simulink model "playback_data"  (R2015a)
settings: Solver=FixedStepDiscrete  SolverMode=SingleTasking  StartTime=76  StopTime=110  FixedStep=sample_time  RelTol=1e-3
undefined symbols (not defined in the file): A1_notch_f1, A2_notch_f1, A_kalman_swing_load, A_kalman_transverse, A_kalman_vertical, A_lpf_accelerometer, A_lpf_dtau, A_lpf_fourbar_angles, A_lpf_imu, A_lpf_lateral_angle, B1_lpf_accelerometer, B1_lpf_dtau, B1_lpf_fourbar_angles, B1_lpf_imu, B1_lpf_lateral_angle, B1_notch_f1, B2_lpf_accelerometer, B2_lpf_dtau, B2_lpf_fourbar_angles, B2_lpf_imu, B2_lpf_lateral_angle, B2_notch_f1, B_dx_versus_x0, B_kalman_swing_load, B_kalman_transverse, B_kalman_vertical, backwards_K_sag_of_t, backwards_P_sag_of_t, C_kalman_swing_load, C_kalman_transverse, C_kalman_vertical, com_leg_motor, com_torso, contact_threshold, control_start_time, d_ankle_to_foot, d_vertical_com, desired_com_forward_velocity, desired_com_lateral_velocity, desired_initial_leg_roll_left, desired_initial_leg_roll_right, desired_stance_beta2, desired_standing_torso_pitch, desired_standing_torso_roll, desired_standing_z, desired_torso_pitch, desired_torso_roll, Discrete, enable_bouncing, fcut_contact, fdesignblkfcn, forward_dx_of_dxstar, forward_x_of_dxstar, g, gcbh, HIP_MTR_MAX_CONT_TORQUE, HIP_MTR_MAX_TORQUE, i_leg_motor, i_robot, i_torso ... (+78)
libraries: simulink x65, dsparch4 x18, ctrlSharedLib x14, dspfdesign x4
(part 5 of 13)

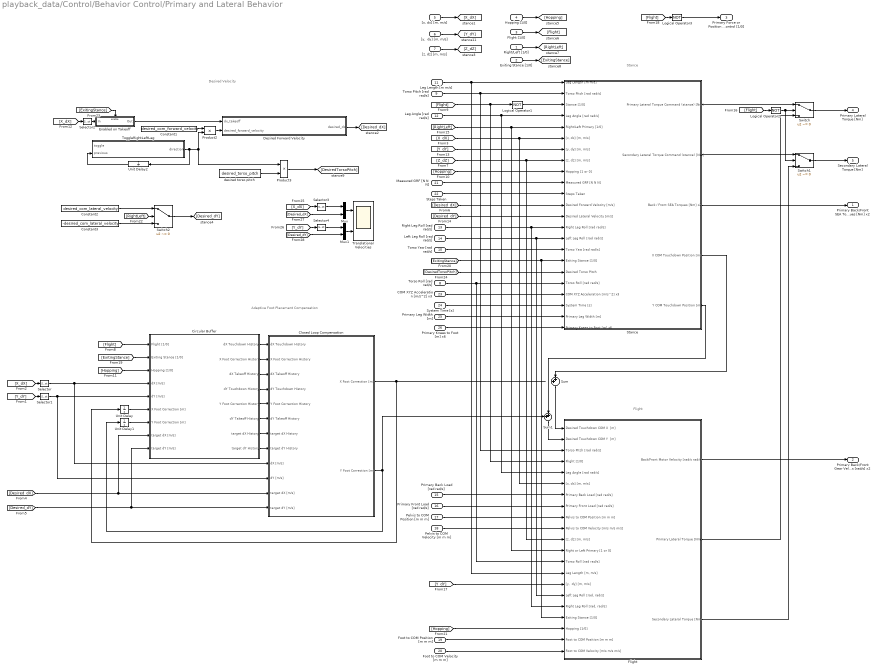
== system playback_data/Control/Behavior Control/Primary and Lateral Behavior ==
  note: Stance
  note: Flight
  note: Adaptive Foot Placement Compensation
  note: Desired Velocity
  Right/Left [1/0] : Inport
  Exiting Stance [1/0] : Inport  Port=2
  Flight [1/0] : Inport  Port=3
  Hopping [1/0] : Inport  Port=4
  "[x, dx] [m, m/s]" : Inport  Port=5
  "[y,  dy] [m, m/s]" : Inport  Port=6
  "[z, dz] [m, m/s]" : Inport  Port=7
  Torso Roll [rad rad/s] : Inport  Port=8
  Torso Pitch [rad rad/s] : Inport  Port=9
  Torso Yaw [rad rad/s] : Inport  Port=10
  Leg Length [m m/s] : Inport  Port=11
  Leg Angle [rad rad/s] : Inport  Port=12
  Right Leg Roll [rad rad/s] : Inport  Port=13
  Left Leg Roll [rad rad/s] : Inport  Port=14
  Primary Back Load [rad rad/s] : Inport  Port=15
  Primary Front Load [rad rad/s] : Inport  Port=16
  Pelvis to COM Position [m m m] : Inport  Port=17
  Pelvis to COM Velocity [m m m] : Inport  Port=18
  Foot to COM Position [m m m] : Inport  Port=19
  Foot to COM Velocity [m m m] : Inport  Port=20
  Measured GRF [N N N] : Inport  Port=21
  Steps Taken : Inport  Port=22
  COM XYZ Acceleration [m/s^2] x3 : Inport  Port=23
  System Time [s] : Inport  Port=24
  Primary Leg Width [m] : Inport  Port=25
  Primary Knees to Foot [m] x6 : Inport  Port=26
  Circular Buffer : Subsystem
  Closed Loop Compensation : Subsystem
  Constant1 : Constant  Value=desired_com_forward_velocity
  Constant2 : Constant  Value=desired_com_lateral_velocity
  Constant3 : Constant  Value=-desired_com_lateral_velocity
  Desired Forward Velocity : MATLAB Function  TreatAsAtomicUnit=on
  Enabled on Takeoff : Subsystem  TreatAsAtomicUnit=on
  Flight : Subsystem
  Logical Operator1 : Logic  Operator=NOT  AllPortsSameDT=off  OutDataTypeStr=boolean
  Logical Operator2 : Logic  Operator=NOT  AllPortsSameDT=off  OutDataTypeStr=boolean
  Logical Operator3 : Logic  Operator=NOT  AllPortsSameDT=off  OutDataTypeStr=boolean
  Mux : Mux  Inputs=2
  Mux1 : Mux  Inputs=2
  Product2 : Product
  Product3 : Product
  Selector{,1..4} (5 alike) : Selector  InputPortWidth=2  Indices=[2]
  Stance : Subsystem
  Sum : Sum  Inputs=++|
  Sum1 : Sum  Inputs=++|
  Switch : Switch  Criteria=u2 ~= 0
  Switch1 : Switch  Criteria=u2 ~= 0
  Switch2 : Switch  Criteria=u2 ~= 0
  ToggleRightLeftLeg : MATLAB Function  TreatAsAtomicUnit=on
      settings: MinAlgLoopOccurrences=on
  Translational Velocities : Scope  NumInputPorts=2
      settings: YMin=-1000~-5  YMax=1000~5  SaveName=ScopeData2  SampleInput=on
  Unit Delay : UnitDelay  SampleTime=-1
  Unit Delay1 : UnitDelay  SampleTime=-1
  Unit Delay2 : UnitDelay  InitialCondition=1  SampleTime=sample_time
  desired torso pitch : Constant  Value=desired_torso_pitch
  Primary Back/Front SEA Torques [Nm] x2 : Outport
  Primary Back/Front Gear Velocities [rad/s] x2 : Outport  Port=2
  Primary Force or Position Control [1/0] : Outport  Port=3  OutDataTypeStr=boolean
  Primary Lateral Torque [Nm] : Outport  Port=4
  Secondary Lateral Torque [Nm] : Outport  Port=5
  wires:
  Leg Length [m m/s]/1 -> Stance/1(Leg Length [m m/s]), Flight/14("Leg Length [m, m/s]")
  Torso Pitch [rad rad/s]/1 -> Stance/2(Torso Pitch [rad rad/s]), Flight/3(Torso Pitch [rad rad/s])
  [Hopping] -> Stance/9(Hopping [1 or 0])
  [X_dX] -> Flight/6("[x, dx] [m, m/s]"), Stance/6("[x, dx] [m, m/s]")
  [RightLeft] -> Flight/12(Right or Left Primary [1 or 0]), Stance/5(Right/Left Primary [1/0])
  Primary Back Load [rad rad/s]/1 -> Flight/7(Primary Back Load [rad rad/s])
  Primary Front Load [rad rad/s]/1 -> Flight/8(Primary Front Load [rad rad/s])
  Leg Angle [rad rad/s]/1 -> Flight/5(Leg Angle [rad rad/s]), Stance/4(Leg Angle [rad rad/s])
  Flight/1(Back/Front Motor Velocity [rad/s rad/s]) -> Primary Back/Front Gear Velocities [rad/s] x2/1
  Logical Operator1/1 -> Stance/3(Stance [1/0])
  [Flight] -> Circular Buffer/1(Flight [1/0])
  Pelvis to COM Position [m m m]/1 -> Flight/9(Pelvis to COM Position [m m m])
  [Z_dZ] -> Stance/8("[z, dz] [m, m/s]"), Flight/11("[z, dz] [m, m/s]")
  Pelvis to COM Velocity [m m m]/1 -> Flight/10(Pelvis to COM Velocity [m/s m/s m/s])
  Torso Roll [rad rad/s]/1 -> Flight/13(Torso Roll [rad rad/s]), Stance/19(Torso Roll [rad rad/s])
  Measured GRF [N N N]/1 -> Stance/10(Measured GRF [N N N])
  Steps Taken/1 -> Stance/11(Steps Taken)
  [Y_dY] -> Flight/15("[y,  dy] [m, m/s]")
  Circular Buffer/1("dX Touchdown History ") -> Closed Loop Compensation/1(dX Touchdown History)
  Circular Buffer/2(X Foot Correction History) -> Closed Loop Compensation/2(X Foot Correction History)
  Circular Buffer/3(dX Takeoff History) -> Closed Loop Compensation/3(dX Takeoff History)
  Circular Buffer/4("dY Touchdown History ") -> Closed Loop Compensation/4(dY Touchdown History)
  Circular Buffer/5(Y Foot Correction History) -> Closed Loop Compensation/5(Y Foot Correction History)
  Circular Buffer/6(dY Takeoff History) -> Closed Loop Compensation/6(dY Takeoff History)
  Circular Buffer/8(target dY History) -> Closed Loop Compensation/8(target dY History)
  Circular Buffer/7(target dX History) -> Closed Loop Compensation/7(target dX History)
  [Desired_dX] -> Circular Buffer/8(target dX [m/s]), Closed Loop Compensation/11(target dX [m/s])
  [Desired_dY] -> Circular Buffer/9(target dY [m/s]), Closed Loop Compensation/12("target dY [m/s] ")
  Stance/4(X COM Touchdown Position [m]) -> Sum/2
  Sum/1 -> Flight/1(Desired Touchdown COM X  [m])
  Closed Loop Compensation/1(X Foot Correction [m]) -> Unit Delay/1
  Selector1/1 -> Circular Buffer/5(dY [m/s]), Closed Loop Compensation/10(dY [m/s])
  Selector/1 -> Circular Buffer/4(dX [m/s]), Closed Loop Compensation/9(dX [m/s])
  Unit Delay1/1 -> Circular Buffer/7(Y Foot Correction [m])
  Unit Delay/1 -> Circular Buffer/6(X Foot Correction [m])
  Closed Loop Compensation/2(Y Foot Correction [m]) -> Unit Delay1/1, Sum1/1
  "[x, dx] [m, m/s]"/1 -> [X_dX]
  "[z, dz] [m, m/s]"/1 -> [Z_dZ]
  "[y,  dy] [m, m/s]"/1 -> [Y_dY]
  [X_dX] -> Selector/1
  [Y_dY] -> Selector1/1
  [Desired_dX] -> Stance/12(Desired Forward Velocity [m/s])
  Flight [1/0]/1 -> [Flight]
  [Flight] -> Flight/4(Flight [1/0]), Logical Operator1/1
  Hopping [1/0]/1 -> [Hopping]
  Stance/5(Y COM Touchdown Position [m]) -> Sum1/2
  Sum1/1 -> Flight/2(Desired Touchdown COM Y  [m])
  Right Leg Roll [rad rad/s]/1 -> Flight/17("Right Leg Roll [rad, rad/s]"), Stance/14(Right Leg Roll [rad rad/s])
  Left Leg Roll [rad rad/s]/1 -> Flight/16("Left Leg Roll [rad, rad/s]"), Stance/15(Left Leg Roll [rad rad/s])
  [Y_dY] -> Stance/7("[y, dy] [m, m/s]")
  [Desired_dY] -> Stance/13(Desired Lateral Velocity [m/s])
  Right/Left [1/0]/1 -> [RightLeft]
  Logical Operator2/1 -> Switch1/2, Switch/2
  Flight/2(Primary Lateral Torque [Nm]) -> Switch/3
  Flight/3(Secondary Lateral Torque [Nm]) -> Switch1/3
  [Flight] -> Logical Operator2/1
  Switch/1 -> Primary Lateral Torque [Nm]/1
  Switch1/1 -> Secondary Lateral Torque [Nm]/1
  [Flight] -> Logical Operator3/1
  Logical Operator3/1 -> Primary Force or Position Control [1/0]/1
  Torso Yaw [rad rad/s]/1 -> Stance/16(Torso Yaw [rad rad/s])
  [Hopping] -> Circular Buffer/3(Hopping [1/0])
  [ExitingStance] -> Circular Buffer/2(Exiting Stance [1/0])
  Exiting Stance [1/0]/1 -> [ExitingStance]
  [ExitingStance] -> Flight/18(Exiting Stance [1/0]), Stance/17(Exiting Stance [1/0])
  [Hopping] -> Flight/19(Hopping [1/0])
  [X_dX] -> Selector2/1
  Switch2/1 -> [Desired_dY]
  Enabled on Takeoff/1(Out) -> Desired Forward Velocity/1(dx_takeoff)
  [RightLeft] -> Switch2/2
  Constant2/1 -> Switch2/1
  Constant3/1 -> Switch2/3
  [ExitingStance] -> Enabled on Takeoff/Enable
  Selector2/1 -> Enabled on Takeoff/1(In)
  Desired Forward Velocity/1(desired_dx) -> [Desired_dX]
  Product2/1 -> Desired Forward Velocity/2(desired_forward_velocity)
  ToggleRightLeftLeg/1(direction) -> Product2/2, Product3/1, Unit Delay2/1
  Unit Delay2/1 -> ToggleRightLeftLeg/2(previous)
  Constant1/1 -> Product2/1
  desired torso pitch/1 -> Product3/2
  Product3/1 -> [DesiredTorsoPitch]
  [DesiredTorsoPitch] -> Stance/18(Desired Torso Pitch)
  Foot to COM Position [m m m]/1 -> Flight/20(Foot to COM Position [m m m])
  Foot to COM Velocity [m m m]/1 -> Flight/21(Foot to COM Velocity [m/s m/s m/s])
  [X_dX] -> Selector3/1
  Selector3/1 -> Mux/1
  [Y_dY] -> Selector4/1
  Selector4/1 -> Mux1/1
  Mux/1 -> Translational Velocities/1
  Mux1/1 -> Translational Velocities/2
  [Desired_dY] -> Mux1/2
  [Desired_dX] -> Mux/2
  COM XYZ Acceleration [m/s^2] x3/1 -> Stance/20(COM XYZ Acceleration [m/s^2] x3)
  System Time [s]/1 -> Stance/21(System Time [s])
  Primary Leg Width [m]/1 -> Stance/22(Primary Leg Width [m])
  Stance/2(Secondary Lateral Torque Command (stance) [Nm]) -> Switch1/1
  Stance/3(Back / Front SEA Torques [Nm] x2) -> Primary Back/Front SEA Torques [Nm] x2/1
  Stance/1(Primary Lateral Torque Command (stance) [Nm]) -> Switch/1
  Primary Knees to Foot [m] x6/1 -> Stance/23(Primary Knees to Foot [m] x6)

== system playback_data/Control/Behavior Control/R Leg Calculator ==
  Front [rad rad/s] : Inport
  Back [rad rad/s] : Inport  Port=2
  Constant : Constant  Value=d_ankle_to_foot-0.01
  Demux1 : Demux  Outputs=2
  Gain1 : Gain  Gain=2*l_seg
  Gain2 : Gain  Gain=l_seg
  Gain3 : Gain  Gain=-1
  Gain4 : Gain  Gain=0.5
  Gain5 : Gain  Gain=0.5
  Gain6 : Gain  Gain=2
  Mux1 : Mux  Inputs=2
  Product : Product  RndMeth=Zero
  Sum : Sum  Inputs=++|
  Sum4 : Sum  Inputs=+|+
  Sum5 : Sum  Inputs=+|-
  Trigonometric Function : Trigonometry  Operator=cos
  Trigonometric Function1 : Trigonometry
  "Leg Length [m m/s] " : Outport
  Leg Angle [rad rad/s] : Outport  Port=2
  Leg Splay [rad rad/s] : Outport  Port=3
  w [m] : Outport  Port=4
  wires:
  Constant/1 -> Sum/1
  Sum/1 -> Mux1/1
  Gain6/1 -> w [m]/1
  Gain4/1 -> Trigonometric Function1/1, Trigonometric Function/1
  Trigonometric Function/1 -> Gain1/1
  Gain1/1 -> Sum/2
  Trigonometric Function1/1 -> Gain2/1
  Product/1 -> Mux1/2
  Front [rad rad/s]/1 -> Sum5/2, Sum4/2
  Back [rad rad/s]/1 -> Sum4/1, Sum5/1
  Demux1/2 -> Gain3/1
  Gain3/1 -> Product/2
  Demux1/1 -> Gain4/1
  Gain2/1 -> Product/1, Gain6/1
  Sum5/1 -> Leg Splay [rad rad/s]/1, Demux1/1
  Mux1/1 -> "Leg Length [m m/s] "/1
  Sum4/1 -> Gain5/1
  Gain5/1 -> Leg Angle [rad rad/s]/1

== system playback_data/Control/Behavior Control/Secondary Leg Behavior ==
  note: Mirror the primary
      | leg motion
  note: Position control the
      | individual four bar segments
  note: Convert to
      | four-bar angles
  Secondary Back Load [rad rad/s] : Inport
  Secondary Front Load [rad rad/s] : Inport  Port=2
  Torso Pitch [rad rad/s] : Inport  Port=3
  Primary Leg Angle [rad rad/s] : Inport  Port=4
  Primary Leg Length [m m/s] : Inport  Port=5
  Avoid Hitting Mechanical Limits : MATLAB Function  TreatAsAtomicUnit=on
  Back/Front PD : Subsystem
  Constant4 : Constant  Value=0
  Demux{1..3,5} (4 alike) : Demux  Outputs=2
  Demux6 : Demux  Outputs=6
  Fcn2 : Fcn  Expr=2*pi-u(1)
  Lowpass Filter (Swing) : Subsystem  DialogController=fdesignblkfcn  InitFcn=fdesignblkfcn(gcbh, {'InitFcn'});  mask(Lowpass Filter){}
      mask help: Design a lowpass filter
      settings: CopyFcn=fdesignblkfcn(gcbh, {'CopyFcn'});
      mask Help: helpview(mapfilelocation('dsp'), 'dsplowpassfilter');
      mask Display: disp('Lowpass')
  Mirrored Leg Length Target : MATLAB Function  TreatAsAtomicUnit=on
  Mux{1..4,7,11} (6 alike) : Mux  Inputs=2
  Mux5 : Mux  Inputs=3
  Mux6 : Mux  Inputs=3
  Sum : Sum  Inputs=++|
  Terminator : Terminator
  Virtual Leg to Four Bar : MATLAB Function  TreatAsAtomicUnit=on
  k_virtual1 : Gain  Gain=2
  k_virtual6 : Gain  Gain=-1
  Secondary Back/Front Motor Torque [Nm Nm] : Outport
  wires:
  Demux5/1 -> Fcn2/1
  Mirrored Leg Length Target/2(dl_leg) -> Mux5/2
  Mirrored Leg Length Target/3(ddl_leg) -> Mux5/3
  Mirrored Leg Length Target/1(l_leg) -> Mux5/1
  Constant4/1 -> Mux6/3
  k_virtual6/1 -> Mux6/2
  Fcn2/1 -> Mux6/1
  Mux7/1 -> Demux6/1
  Virtual Leg to Four Bar/1(back) -> Avoid Hitting Mechanical Limits/1(back_desired)
  Virtual Leg to Four Bar/2(dback) -> Avoid Hitting Mechanical Limits/2(dback_desired)
  Virtual Leg to Four Bar/3(ddback) -> Avoid Hitting Mechanical Limits/3(ddback_desired)
  Virtual Leg to Four Bar/4(front) -> Avoid Hitting Mechanical Limits/4(front_desired)
  Virtual Leg to Four Bar/5(dfront) -> Avoid Hitting Mechanical Limits/5(dfront_desired)
  Virtual Leg to Four Bar/6(ddfront) -> Avoid Hitting Mechanical Limits/6(ddfront_desired)
  Demux6/1 -> Virtual Leg to Four Bar/1(l_leg)
  Demux6/2 -> Virtual Leg to Four Bar/2(dl_leg)
  Demux6/3 -> Virtual Leg to Four Bar/3(ddl_leg)
  Demux6/4 -> Virtual Leg to Four Bar/4(phi)
  Demux6/5 -> Virtual Leg to Four Bar/5(dphi)
  Demux6/6 -> Virtual Leg to Four Bar/6(ddphi)
  Mux11/1 -> Back/Front PD/4(Measured Velocity [rad/s] [back front])
  Demux2/2 -> Mux11/2
  Mux4/1 -> Back/Front PD/3(Measured Position [rad] [back front])
  Mux1/1 -> Back/Front PD/1(Desired Position [rad] [back front])
  Demux3/2 -> Mux11/1
  Demux3/1 -> Mux4/1
  Avoid Hitting Mechanical Limits/2(front_cmd) -> Mux1/2
  Avoid Hitting Mechanical Limits/1(back_cmd) -> Mux1/1
  Demux2/1 -> Mux4/2
  Secondary Front Load [rad rad/s]/1 -> Demux2/1
  Secondary Back Load [rad rad/s]/1 -> Demux3/1
  Avoid Hitting Mechanical Limits/3(dback_cmd) -> Mux2/1
  Avoid Hitting Mechanical Limits/4(dfront_cmd) -> Mux2/2
  Avoid Hitting Mechanical Limits/5(ddback_cmd) -> Mux3/1
  Avoid Hitting Mechanical Limits/6(ddfront_cmd) -> Mux3/2
  Mux2/1 -> Back/Front PD/2(Desired Velocity [rad/s] [back front])
  Primary Leg Angle [rad rad/s]/1 -> Sum/2
  Demux1/1 -> Mirrored Leg Length Target/1(primary_l_leg)
  Demux1/2 -> Mirrored Leg Length Target/2(primary_dl_leg)
  Primary Leg Length [m m/s]/1 -> Demux1/1
  Sum/1 -> Demux5/1
  Torso Pitch [rad rad/s]/1 -> k_virtual1/1
  k_virtual1/1 -> Sum/1
  Mux5/1 -> Mux7/1
  Mux3/1 -> Terminator/1
  Demux5/2 -> k_virtual6/1
  Mux6/1 -> Mux7/2
  Back/Front PD/1(Commanded Velocity [rad/s] [back front]) -> Lowpass Filter (Swing)/1(In)
  Lowpass Filter (Swing)/1(Out) -> Secondary Back/Front Motor Torque [Nm Nm]/1

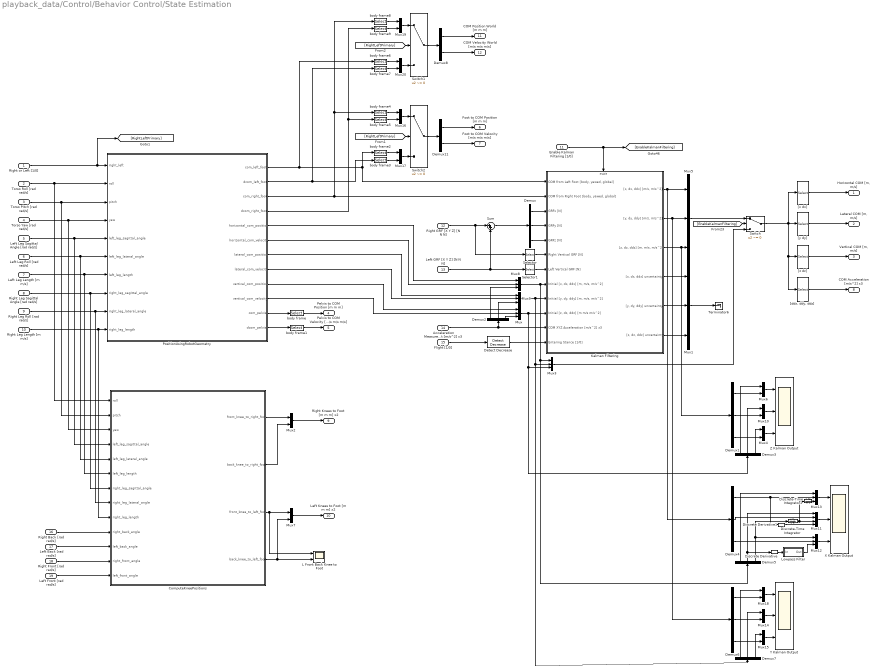
== system playback_data/Control/Behavior Control/State Estimation ==
  Right or Left [1/0] : Inport
  Torso Roll [rad rad/s] : Inport  Port=2
  Torso Pitch [rad rad/s] : Inport  Port=3
  Torso Yaw [rad rad/s] : Inport  Port=4
  Left Leg Sagittal Angle [rad rad/s] : Inport  Port=5
  Left Leg Roll [rad rad/s] : Inport  Port=6
  Left Leg Length [m m/s] : Inport  Port=7
  Right Leg Sagittal Angle [rad rad/s] : Inport  Port=8
  Right Leg Roll [rad rad/s] : Inport  Port=9
  Right Leg Length [m m/s] : Inport  Port=10
  Enable Kalman Filtering [1/0] : Inport  Port=11
  Right GRF [X Y Z] [N N N] : Inport  Port=12
  Left GRF [X Y Z] [N N N] : Inport  Port=13
  " Acceleration Measurement [m/s^2] x3" : Inport  Port=14
  Flight [1/0] : Inport  Port=15
  Right Back [rad rad/s] : Inport  Port=16
  Left Back [rad rad/s] : Inport  Port=17
  Right Front [rad rad/s] : Inport  Port=18
  Left Front [rad rad/s] : Inport  Port=19
  ComputeKneePositions : MATLAB Function  TreatAsAtomicUnit=on
  Demux{,1..7} (8 alike) : Demux  Outputs=3
  Demux11 : Demux  Outputs=2
  Demux8 : Demux  Outputs=2
  Detect Decrease : simulink/Logic and Bit Operations/Detect Decrease  vinit=0.0  InputProcessing=Inherited  OutDataTypeStr=boolean
  Discrete Derivative : simulink/Discrete/Discrete Derivative  gainval=1.0  ICPrevScaledInput=0.0  InputProcessing=Inherited  OutMin=[]  OutMax=[]  OutDataType=fixdt(1, 16)  OutScaling=2^-10  DoSatur=off
  Discrete Derivative1 : simulink/Discrete/Discrete Derivative  gainval=1.0  ICPrevScaledInput=0.0  InputProcessing=Inherited  OutMin=[]  OutMax=[]  OutDataType=fixdt(1, 16)  OutScaling=2^-10  DoSatur=off
  Discrete-Time Integrator : DiscreteIntegrator  InitialConditionSetting=State (most efficient)  SampleTime=-1
  Discrete-Time Integrator1 : DiscreteIntegrator  InitialConditionSetting=State (most efficient)  SampleTime=-1
  Kalman Filtering : Subsystem
  L Front Back Knee to Foot : Scope  NumInputPorts=2
      settings: YMin=-0.425~-0.5  YMax=-0.025~0.3  SaveName=ScopeData44  SampleInput=on
  Lowpass Filter : Subsystem  DialogController=fdesignblkfcn  InitFcn=fdesignblkfcn(gcbh, {'InitFcn'});  mask(Lowpass Filter){}
      mask help: Design a lowpass filter
      settings: CopyFcn=fdesignblkfcn(gcbh, {'CopyFcn'});
      mask Help: helpview(mapfilelocation('dsp'), 'dsplowpassfilter');
      mask Display: disp('Lowpass')
  Mux{,1,3,5,8..9,12..13} (8 alike) : Mux  Inputs=3
  Mux{2,4,6..7,10,14..20} (12 alike) : Mux  Inputs=2
  Mux11 : Mux
  PositionUsingRobotGeometry : MATLAB Function  TreatAsAtomicUnit=on
  Selector : Selector  InputPortWidth=3  Indices=[3]
  Selector1 : Selector  InputPortWidth=3  Indices=[3]
  Sum : Sum  Inputs=|++
  Switch : Switch  Criteria=u2 ~= 0
  Switch1 : Switch  Criteria=u2 ~= 0
  Switch2 : Switch  Criteria=u2 ~= 0
  Terminator6 : Terminator
  X Kalman Output : Scope  NumInputPorts=3
      settings: TimeRange=3.774467455621291  YMin=5.55112e-17~-0.075~-0.5  YMax=2.1~0.25~0.6  SaveName=ScopeData29  SampleInput=on
  Y Kalman Output : Scope  NumInputPorts=3
      settings: TimeRange=39.999  YMin=0.05~-0.7~-2  YMax=0.18~1.1~3.5  SaveName=ScopeData30  SampleInput=on
  Z Kalman Output : Scope  NumInputPorts=3
      settings: TimeRange=3.175000000000004  YMin=0~-0.04~-0.7  YMax=0.9~0.035~0.6  SaveName=ScopeData27  SampleInput=on
  "[ddx, ddy, ddz]" : Selector  InputPortWidth=9  Indices=[3 6 9]
  "[x dx]" : Selector  InputPortWidth=9  Indices=[1 2]
  "[y dy]" : Selector  InputPortWidth=9  Indices=[4 5]
  "[z dz]" : Selector  InputPortWidth=9  Indices=[7 8]
  body frame : Selector  InputPortWidth=9  Indices=[1 2 3]
  body frame1 : Selector  InputPortWidth=9  Indices=[1 2 3]
  body frame{2..5} (4 alike) : Selector  InputPortWidth=9  Indices=[4 5 6]
  body frame{6..9} (4 alike) : Selector  InputPortWidth=9  Indices=[7 8 9]
  "Horizontal COM [m, m/s]" : Outport
  "Lateral COM [m, m/s]" : Outport  Port=2
  "Vertical COM [m, m/s]" : Outport  Port=3
  Pelvis to COM Position [m m m] : Outport  Port=4
  Pelvis to COM Velocity [m/s m/s m/s] : Outport  Port=5
  Foot to COM Position [m m m] : Outport  Port=6
  Foot to COM Velocity [m/s m/s m/s] : Outport  Port=7
  COM Acceleration [m/s^2] x3 : Outport  Port=8
  Right Knees to Foot [m m m] x2 : Outport  Port=9
  Left Knees to Foot [m m m] x2 : Outport  Port=10
  COM Position World [m m m] : Outport  Port=11  PortDimensions=3
  COM Velocity World [m/s m/s m/s] : Outport  Port=12  PortDimensions=3
  wires:
  Discrete-Time Integrator1/1 -> Mux13/3
  Lowpass Filter/1(Out) -> Mux12/3
  Discrete Derivative/1 -> Lowpass Filter/1(In)
  Discrete-Time Integrator/1 -> Discrete-Time Integrator1/1, Mux11/3
  Demux5/3 -> Mux12/1, Discrete-Time Integrator/1
  Demux5/2 -> Mux11/1, Discrete Derivative/1
  Demux5/1 -> Mux13/1
  Demux4/3 -> Mux12/2
  Mux11/1 -> X Kalman Output/2
  Demux4/1 -> Discrete Derivative1/1, Mux13/2
  Demux4/2 -> Mux11/2
  Mux13/1 -> X Kalman Output/1
  Mux12/1 -> X Kalman Output/3
  Mux9/1 -> Mux3/2, Demux7/1, Kalman Filtering/9("Initial [y, dy, ddy] [m, m/s, m/s^2]")
  Mux8/1 -> Mux3/1, Demux5/1, Kalman Filtering/8("Initial [x, dx, ddx] [m, m/s, m/s^2]")
  "[ddx, ddy, ddz]"/1 -> COM Acceleration [m/s^2] x3/1
  Mux3/1 -> Switch/3
  Demux2/2 -> Mux9/3
  Demux2/1 -> Mux8/3
  Demux2/3 -> Mux/3
  " Acceleration Measurement [m/s^2] x3"/1 -> Demux2/1, Kalman Filtering/11(COM XYZ Acceleration [m/s^2] x3)
  PositionUsingRobotGeometry/5(horizontal_com_position) -> Mux8/1
  Left Leg Sagittal Angle [rad rad/s]/1 -> PositionUsingRobotGeometry/5(left_leg_sagittal_angle), ComputeKneePositions/4(left_leg_sagittal_angle)
  Left Leg Roll [rad rad/s]/1 -> PositionUsingRobotGeometry/6(left_leg_lateral_angle), ComputeKneePositions/5(left_leg_lateral_angle)
  Left Leg Length [m m/s]/1 -> PositionUsingRobotGeometry/7(left_leg_length), ComputeKneePositions/6(left_leg_length)
  Right Leg Sagittal Angle [rad rad/s]/1 -> PositionUsingRobotGeometry/8(right_leg_sagittal_angle), ComputeKneePositions/7(right_leg_sagittal_angle)
  Right Leg Roll [rad rad/s]/1 -> ComputeKneePositions/8(right_leg_lateral_angle), PositionUsingRobotGeometry/9(right_leg_lateral_angle)
  Right Leg Length [m m/s]/1 -> ComputeKneePositions/9(right_leg_length), PositionUsingRobotGeometry/10(right_leg_length)
  Right or Left [1/0]/1 -> [RightLeftPrimary], PositionUsingRobotGeometry/1(right_left)
  Torso Roll [rad rad/s]/1 -> PositionUsingRobotGeometry/2(roll), ComputeKneePositions/1(roll)
  Torso Yaw [rad rad/s]/1 -> PositionUsingRobotGeometry/4(yaw), ComputeKneePositions/3(yaw)
  Torso Pitch [rad rad/s]/1 -> PositionUsingRobotGeometry/3(pitch), ComputeKneePositions/2(pitch)
  Mux5/1 -> Switch/1
  Selector/1 -> Kalman Filtering/6(Right Vertical GRF [N])
  Selector1/1 -> Kalman Filtering/7(Left Vertical GRF [N])
  Left GRF [X Y Z] [N N N]/1 -> Selector1/1, Sum/2
  Right GRF [X Y Z] [N N N]/1 -> Selector/1, Sum/1
  Sum/1 -> Demux/1
  Enable Kalman Filtering [1/0]/1 -> Kalman Filtering/Enable, [EnableKalmanFiltering]
  Demux/1 -> Kalman Filtering/3(GRFx [N])
  Mux1/1 -> Terminator6/1
  PositionUsingRobotGeometry/12(dcom_pelvis) -> body frame1/1
  PositionUsingRobotGeometry/11(com_pelvis) -> body frame/1
  "[x dx]"/1 -> "Horizontal COM [m, m/s]"/1
  body frame/1 -> Pelvis to COM Position [m m m]/1
  body frame1/1 -> Pelvis to COM Velocity [m/s m/s m/s]/1
  PositionUsingRobotGeometry/7(lateral_com_position) -> Mux9/1
  "[z dz]"/1 -> "Vertical COM [m, m/s]"/1
  Switch/1 -> "[x dx]"/1, "[y dy]"/1, "[z dz]"/1, "[ddx, ddy, ddz]"/1
  "[y dy]"/1 -> "Lateral COM [m, m/s]"/1
  Demux/3 -> Kalman Filtering/5(GRFz [N])
  Demux/2 -> Kalman Filtering/4(GRFy [N])
  Kalman Filtering/1("[x, dx, ddx] [m/s, m/s^2]") -> Mux5/1, Demux4/1
  Kalman Filtering/3("[z, dz, ddz] [m, m/s, m/s^2]") -> Demux1/1, Mux5/3
  Kalman Filtering/2("[y, dy, ddy] [m/s, m/s^2]") -> Demux6/1, Mux5/2
  Kalman Filtering/5("[y, dy, ddy] uncertainty") -> Mux1/2
  Kalman Filtering/4("[x, dx, ddx] uncertainty") -> Mux1/1
  Kalman Filtering/6("[z, dz, ddz] uncertainty") -> Mux1/3
  PositionUsingRobotGeometry/9(vertical_com_position) -> Mux/1
  PositionUsingRobotGeometry/10(vertical_com_velocity) -> Mux/2
  Mux/1 -> Mux3/3, Demux3/1, Kalman Filtering/10("Initial [z, dz, ddz] [m m/s m/s^2]")
  PositionUsingRobotGeometry/8(lateral_com_velocity) -> Mux9/2
  PositionUsingRobotGeometry/6(horizontal_com_velocity) -> Mux8/2
  [RightLeftPrimary] -> Switch2/2
  Mux17/1 -> Switch2/3
  Mux16/1 -> Switch2/1
  Switch2/1 -> Demux11/1
  Demux11/2 -> Foot to COM Velocity [m/s m/s m/s]/1
  Demux11/1 -> Foot to COM Position [m m m]/1
  body frame2/1 -> Mux17/1
  body frame3/1 -> Mux17/2
  body frame5/1 -> Mux16/2
  body frame4/1 -> Mux16/1
  Flight [1/0]/1 -> Detect Decrease/1
  Detect Decrease/1 -> Kalman Filtering/12(Entering Stance [1/0])
  Mux4/1 -> Z Kalman Output/3
  Mux6/1 -> Z Kalman Output/1
  Demux1/2 -> Mux10/2
  Demux1/1 -> Mux6/2
  Mux10/1 -> Z Kalman Output/2
  Demux1/3 -> Mux4/2
  Demux3/1 -> Mux6/1
  Demux3/2 -> Mux10/1
  Demux3/3 -> Mux4/1
  Mux15/1 -> Y Kalman Output/3
  Mux18/1 -> Y Kalman Output/1
  Demux6/2 -> Mux14/2
  Demux6/1 -> Mux18/2
  Mux14/1 -> Y Kalman Output/2
  Demux6/3 -> Mux15/2
  Demux7/1 -> Mux18/1
  Demux7/2 -> Mux14/1
  Demux7/3 -> Mux15/1
  ComputeKneePositions/1(front_knee_to_right_foot) -> Mux2/1
  ComputeKneePositions/2(back_knee_to_right_foot) -> Mux2/2
  ComputeKneePositions/3(front_knee_to_left_foot) -> L Front Back Knee to Foot/1, Mux7/1
  ComputeKneePositions/4(back_knee_to_left_foot) -> L Front Back Knee to Foot/2, Mux7/2
  Mux2/1 -> Right Knees to Foot [m m m] x2/1
  Mux7/1 -> Left Knees to Foot [m m m] x2/1
  Left Front [rad rad/s]/1 -> ComputeKneePositions/13(left_front_angle)
  Right Front [rad rad/s]/1 -> ComputeKneePositions/12(right_front_angle)
  Left Back [rad rad/s]/1 -> ComputeKneePositions/11(left_back_angle)
  Right Back [rad rad/s]/1 -> ComputeKneePositions/10(right_back_angle)
  [EnableKalmanFiltering] -> Switch/2
  PositionUsingRobotGeometry/1(com_left_foot) -> body frame6/1, body frame2/1, Kalman Filtering/1("COM from Left Foot [body, yawed, global]")
  PositionUsingRobotGeometry/2(dcom_left_foot) -> body frame7/1, body frame3/1
  PositionUsingRobotGeometry/3(com_right_foot) -> body frame8/1, body frame4/1, Kalman Filtering/2("COM from Right Foot [body, yawed, global]")
  PositionUsingRobotGeometry/4(dcom_right_foot) -> body frame9/1, body frame5/1
  [RightLeftPrimary] -> Switch1/2
  Mux20/1 -> Switch1/3
  Mux19/1 -> Switch1/1
  Switch1/1 -> Demux8/1
  Demux8/2 -> COM Velocity World [m/s m/s m/s]/1
  Demux8/1 -> COM Position World [m m m]/1
  body frame6/1 -> Mux20/1
  body frame7/1 -> Mux20/2
  body frame9/1 -> Mux19/2
  body frame8/1 -> Mux19/1
  Discrete Derivative1/1 -> Mux11/4

== system playback_data/Control1/Actuator Control with Torque SEA commands/Compare SEA Signals ==
  Desired : Inport
  Measured : Inport  Port=2
  Demux : Demux
  Demux1 : Demux
  Mux{6..9} (4 alike) : Mux  Inputs=2
  RB : Outport
  RF : Outport  Port=2
  LB : Outport  Port=3
  LF : Outport  Port=4
  wires:
  Demux/3 -> Mux8/1
  Demux/2 -> Mux7/1
  Demux1/1 -> Mux6/2
  Demux/1 -> Mux6/1
  Demux/4 -> Mux9/1
  Demux1/4 -> Mux9/2
  Measured/1 -> Demux1/1
  Demux1/2 -> Mux7/2
  Desired/1 -> Demux/1
  Demux1/3 -> Mux8/2
  Mux6/1 -> RB/1
  Mux7/1 -> RF/1
  Mux9/1 -> LF/1
  Mux8/1 -> LB/1

== system playback_data/Control1/Actuator Control with Torque SEA commands/Compare Signals ==
  Measurement : Inport
  Filtered : Inport  Port=2
  Expected : Inport  Port=3
  Demux : Demux
  Demux1 : Demux
  Demux2 : Demux
  Mux{6..9} (4 alike) : Mux  Inputs=3
  RB : Outport
  RF : Outport  Port=2
  LB : Outport  Port=3
  LF : Outport  Port=4
  wires:
  Mux8/1 -> LB/1
  Mux9/1 -> LF/1
  Mux7/1 -> RF/1
  Mux6/1 -> RB/1
  Demux1/3 -> Mux8/2
  Measurement/1 -> Demux/1
  Demux1/2 -> Mux7/2
  Filtered/1 -> Demux1/1
  Demux1/4 -> Mux9/2
  Demux/4 -> Mux9/1
  Demux/1 -> Mux6/1
  Demux1/1 -> Mux6/2
  Demux/2 -> Mux7/1
  Demux/3 -> Mux8/1
  Expected/1 -> Demux2/1
  Demux2/1 -> Mux6/3
  Demux2/2 -> Mux7/3
  Demux2/3 -> Mux8/3
  Demux2/4 -> Mux9/3

== system playback_data/Control1/Actuator Control with Torque SEA commands/Compare Torque Derivative Signals ==
  Measured : Inport
  Filtered : Inport  Port=2
  Expected : Inport  Port=3
  Demux : Demux
  Demux1 : Demux
  Demux2 : Demux
  Mux{6..9} (4 alike) : Mux  Inputs=3
  RB : Outport
  RF : Outport  Port=2
  LB : Outport  Port=3
  LF : Outport  Port=4
  wires:
  Demux2/4 -> Mux9/3
  Demux2/3 -> Mux8/3
  Demux2/2 -> Mux7/3
  Demux2/1 -> Mux6/3
  Expected/1 -> Demux2/1
  Demux/3 -> Mux8/1
  Demux/2 -> Mux7/1
  Demux1/1 -> Mux6/2
  Demux/1 -> Mux6/1
  Demux/4 -> Mux9/1
  Demux1/4 -> Mux9/2
  Filtered/1 -> Demux1/1
  Demux1/2 -> Mux7/2
  Measured/1 -> Demux/1
  Demux1/3 -> Mux8/2
  Mux6/1 -> RB/1
  Mux7/1 -> RF/1
  Mux9/1 -> LF/1
  Mux8/1 -> LB/1

== system playback_data/Control1/Actuator Control with Torque SEA commands/Compare Velocities ==
  Desired : Inport
  Measured : Inport  Port=2
  Demux : Demux
  Demux1 : Demux
  Mux{6..9} (4 alike) : Mux  Inputs=2
  RB : Outport
  RF : Outport  Port=2
  LB : Outport  Port=3
  LF : Outport  Port=4
  wires:
  Demux1/3 -> Mux8/2
  Desired/1 -> Demux/1
  Demux1/2 -> Mux7/2
  Measured/1 -> Demux1/1
  Demux1/4 -> Mux9/2
  Demux/4 -> Mux9/1
  Demux/1 -> Mux6/1
  Demux1/1 -> Mux6/2
  Demux/2 -> Mux7/1
  Demux/3 -> Mux8/1
  Mux6/1 -> RB/1
  Mux7/1 -> RF/1
  Mux8/1 -> LB/1
  Mux9/1 -> LF/1

== system playback_data/Control1/Actuator Control with Torque SEA commands/Contact Velocities ==
  Contact [1/0] x4 : Inport
  Velocities [rad/s] x4 : Inport  Port=2
  Demux : Demux
  Demux1 : Demux
  Mux : Mux
  Velocity on Contact : Subsystem
  Velocity on Contact1 : Subsystem
  Velocity on Contact2 : Subsystem
  Velocity on Contact3 : Subsystem
  Contact Velocities [rad/s] x4 : Outport
  wires:
  Mux/1 -> Contact Velocities [rad/s] x4/1
  Demux/2 -> Velocity on Contact1/Trigger
  Velocity on Contact/1(out) -> Mux/1
  Contact [1/0] x4/1 -> Demux/1
  Velocity on Contact1/1(out) -> Mux/2
  Demux/3 -> Velocity on Contact2/Trigger
  Demux/4 -> Velocity on Contact3/Trigger
  Demux/1 -> Velocity on Contact/Trigger
  Velocity on Contact3/1(out) -> Mux/4
  Velocity on Contact2/1(out) -> Mux/3
  Velocities [rad/s] x4/1 -> Demux1/1
  Demux1/1 -> Velocity on Contact/1(in)
  Demux1/2 -> Velocity on Contact1/1(in)
  Demux1/3 -> Velocity on Contact2/1(in)
  Demux1/4 -> Velocity on Contact3/1(in)

== system playback_data/Control1/Actuator Control with Torque SEA commands/Desired Torque Derivative ==
  Signal x4 : Inport
  Reset [1/0] x4 : Inport  Port=2
  Demux : Demux
  Demux1 : Demux
  Gain1 : Gain  Gain=1/sample_time
  Logical Operator : Logic  Operator=NOT  AllPortsSameDT=off  OutDataTypeStr=boolean
  Mux : Mux
  Product : Product
  difference : simulink/Discrete/Difference  ICPrevInput=0.0  InputProcessing=Inherited  OutMin=[]  OutMax=[]  OutDataType=fixdt(1, 16)  OutScaling=2^-10  DoSatur=off
  two_pole_filter{,1..3} (4 alike) : DiscreteTransferFcn  Numerator=[A_lpf_dtau 0 0]  Denominator=[1 B1_lpf_dtau B2_lpf_dtau]  ExternalReset=Rising  SampleTime=sample_time
      settings: InputPortMap=u0,r7
  Derivative x4 : Outport
  wires:
  Demux/1 -> two_pole_filter/1
  difference/1 -> Product/1
  Mux/1 -> Derivative x4/1
  Signal x4/1 -> Gain1/1
  Gain1/1 -> difference/1
  Logical Operator/1 -> Product/2
  Reset [1/0] x4/1 -> Demux1/1, Logical Operator/1
  two_pole_filter/1 -> Mux/1
  Product/1 -> Demux/1
  two_pole_filter1/1 -> Mux/2
  two_pole_filter2/1 -> Mux/3
  two_pole_filter3/1 -> Mux/4
  Demux/2 -> two_pole_filter1/1
  Demux/3 -> two_pole_filter2/1
  Demux/4 -> two_pole_filter3/1
  Demux1/1 -> two_pole_filter/2
  Demux1/2 -> two_pole_filter1/2
  Demux1/3 -> two_pole_filter2/2
  Demux1/4 -> two_pole_filter3/2

== system playback_data/Control1/Actuator Control with Torque SEA commands/Expected Forces on Foot ==
  R/L Leg Length [m] x2 : Inport
  R/L Leg Width [m] x2 : Inport  Port=2
  Torques on Load [Nm] x4 : Inport  Port=3
  Divide : Product  Inputs=/*
  Divide1 : Product  Inputs=/*
  Gain3 : Gain  Gain=-1
  Gain6 : Gain  Gain=-1
  Selector2 : Selector  InputPortWidth=4  Indices=[1 3]
  Selector7 : Selector  InputPortWidth=4  Indices=[2 4]
  Sum5 : Sum  Inputs=|-+
  Sum6 : Sum  Inputs=++|
  R/L Orthogonal Force [N] x2 : Outport
  R/L Axial Force [N] x2 : Outport  Port=2
  wires:
  Gain6/1 -> R/L Orthogonal Force [N] x2/1
  Gain3/1 -> R/L Axial Force [N] x2/1
  Sum5/1 -> Divide1/2
  Selector7/1 -> Sum6/2, Sum5/2
  Sum6/1 -> Divide/2
  Selector2/1 -> Sum5/1, Sum6/1
  Divide1/1 -> Gain3/1
  Torques on Load [Nm] x4/1 -> Selector2/1, Selector7/1
  R/L Leg Width [m] x2/1 -> Divide1/1
  R/L Leg Length [m] x2/1 -> Divide/1
  Divide/1 -> Gain6/1

== system playback_data/Control1/Actuator Control with Torque SEA commands/Load Torque Kalman Filter ==
  Measured Spring Torque [Nm] x4 : Inport
  Load Position [rad/s] x4 : Inport  Port=2
  Load Velocity [rad/s] x4 : Inport  Port=3
  Reset [1/0] x4 : Inport  Port=4
  Constant{,1..3} (4 alike) : Constant  Value=P0_kalman_swing_load
  Demux2 : Demux
  Difference{,1..3} (4 alike) : simulink/Discrete/Difference  ICPrevInput=0.0  InputProcessing=Inherited  OutMin=[]  OutMax=[]  OutDataType=fixdt(1, 16)  OutScaling=2^-10  DoSatur=off
  Gain{1..4} (4 alike) : Gain  Gain=1/mean(j_segments)
  Gain5 : Gain  Gain=mean(j_segments)
  MATLAB Function : MATLAB Function  TreatAsAtomicUnit=on
  Mux : Mux
  Mux{1,3,5,7} (4 alike) : Mux  Inputs=2
  Mux{2,4,6,8} (4 alike) : Mux  Inputs=3
  Selector : Selector  InputPortWidth=4  Indices=[1]
  Selector{1..3,12} (4 alike) : Selector  InputPortWidth=3  Indices=[3]
  Selector10 : Selector  InputPortWidth=4  Indices=[2]
  Selector11 : Selector  InputPortWidth=4  Indices=[3]
  Selector13 : Selector  InputPortWidth=4  Indices=[3]
  Selector14 : Selector  InputPortWidth=4  Indices=[4]
  Selector15 : Selector  InputPortWidth=4  Indices=[4]
  Selector4 : Selector  InputPortWidth=4  Indices=[1]
  Selector5 : Selector  InputPortWidth=4  Indices=[1]
  Selector6 : Selector  InputPortWidth=4  Indices=[2]
  Selector7 : Selector  InputPortWidth=4  Indices=[3]
  Selector8 : Selector  InputPortWidth=4  Indices=[4]
  Selector9 : Selector  InputPortWidth=4  Indices=[2]
  Swing Load Kalman Filter{,1..3} (4 alike) : ctrlSharedLib/Kalman Filter  TimeDomain=Discrete-Time  UseCurrentEstimator=on  ModelSource=Individual A, B, C, D matrices  ModelSourceVariable=A_kf  A=A_kalman_swing_load  B=B_kalman_swing_load  C=C_kalman_swing_load  D=0  NumberOfStates=2  NumberOfInputs=1  NumberOfOutputs=2  InitialEstimateSource=Input port  X0=initial_dx_estimate  P0=P0_kalman_transverse  UseK=off  UseGH=on  NumberOfProcessNoiseInputs=1  G=G_kalman_swing_load  TimeInvariantG=on  H=0  TimeInvariantH=on  Q=Q_kalman_SEA_torque_difference  TimeInvariantQ=on  R=1  TimeInvariantR=off  N=0  TimeInvariantN=on  AddInputPort=on  AddEnablePort=off  ExternalReset=Rising  OutputEstimatedY=off  OutputP=off  Ts=sample_time
  Load Torques [Nm] x4 : Outport
  wires:
  Mux6/1 -> Swing Load Kalman Filter/3
  Mux5/1 -> Swing Load Kalman Filter/2
  Difference/1 -> Swing Load Kalman Filter/1
  Demux2/1 -> Gain3/1, Mux5/2, Difference/1
  Swing Load Kalman Filter/1 -> Selector12/1
  Selector12/1 -> Mux/1
  Mux2/1 -> Swing Load Kalman Filter1/3
  Mux1/1 -> Swing Load Kalman Filter1/2
  Difference1/1 -> Swing Load Kalman Filter1/1
  Demux2/2 -> Gain1/1, Mux1/2, Difference1/1
  Gain1/1 -> Mux2/3
  Mux4/1 -> Swing Load Kalman Filter2/3
  Mux3/1 -> Swing Load Kalman Filter2/2
  Difference2/1 -> Swing Load Kalman Filter2/1
  Demux2/3 -> Difference2/1, Mux3/2, Gain2/1
  Gain2/1 -> Mux4/3
  Mux8/1 -> Swing Load Kalman Filter3/3
  Mux7/1 -> Swing Load Kalman Filter3/2
  Difference3/1 -> Swing Load Kalman Filter3/1
  Demux2/4 -> Difference3/1, Mux7/2, Gain4/1
  Gain4/1 -> Mux8/3
  Swing Load Kalman Filter1/1 -> Selector1/1
  Swing Load Kalman Filter3/1 -> Selector3/1
  Swing Load Kalman Filter2/1 -> Selector2/1
  Mux/1 -> Gain5/1
  Selector1/1 -> Mux/2
  Selector2/1 -> Mux/3
  Selector3/1 -> Mux/4
  Reset [1/0] x4/1 -> [Reset]
  Load Velocity [rad/s] x4/1 -> [LoadVelocities]
  Measured Spring Torque [Nm] x4/1 -> MATLAB Function/1(spring_torques), Demux2/1
  Gain5/1 -> Load Torques [Nm] x4/1
  Gain3/1 -> Mux6/3
  Load Position [rad/s] x4/1 -> [LoadPositions]
  [LoadPositions] -> Selector/1
  [LoadVelocities] -> Selector4/1
  Selector/1 -> Mux6/1, Mux5/1
  Selector4/1 -> Mux6/2
  [Reset] -> Selector5/1
  Selector5/1 -> Swing Load Kalman Filter/5
  [Reset] -> Selector6/1
  Selector6/1 -> Swing Load Kalman Filter1/5
  [Reset] -> Selector7/1
  Selector7/1 -> Swing Load Kalman Filter2/5
  [Reset] -> Selector8/1
  Selector8/1 -> Swing Load Kalman Filter3/5
  [LoadVelocities] -> Selector9/1
  [LoadPositions] -> Selector10/1
  [LoadVelocities] -> Selector11/1
  [LoadPositions] -> Selector13/1
  [LoadVelocities] -> Selector14/1
  [LoadPositions] -> Selector15/1
  Selector15/1 -> Mux8/1, Mux7/1
  Selector13/1 -> Mux4/1, Mux3/1
  Selector11/1 -> Mux4/2
  Selector14/1 -> Mux8/2
  Selector9/1 -> Mux2/2
  Selector10/1 -> Mux2/1, Mux1/1
  Constant/1 -> Swing Load Kalman Filter1/4
  MATLAB Function/1(R1) -> [R1]
  MATLAB Function/2(R2) -> [R2]
  MATLAB Function/3(R3) -> [R3]
  MATLAB Function/4(R4) -> [R4]
  [R2] -> Swing Load Kalman Filter1/6
  [R1] -> Swing Load Kalman Filter/6
  Constant1/1 -> Swing Load Kalman Filter/4
  [R3] -> Swing Load Kalman Filter2/6
  Constant2/1 -> Swing Load Kalman Filter2/4
  Constant3/1 -> Swing Load Kalman Filter3/4
  [R4] -> Swing Load Kalman Filter3/6

== system playback_data/Control1/Actuator Control with Torque SEA commands/Lowpass Filter ==
  In : Inport
  Generated Filter Block : dsparch4/Biquad Filter  Tag=BlockMethodSubSystem  IIRFiltStruct=Direct form II  CoeffSource=Specify via dialog  BiQuadCoeffs=[1.0054190789171848 -2 1.0054190789171853 1 -1.9557970115108714 0.95685429506963915]  a0Flag=Warning  IC=0  ICnum=0  ICden=0  denAccumFracLength=30  denProdOutputFracLength=30  secondMemoryFracLength=15  roundingMode=Floor  overflowMode=off  ScaleValues=[0.0010519560093213882;92.733879468734756]  optimizeScaleValues=off  ScaleValueMode=Specify via input port (g)  scaleValueFracLength=14  FilterSource=Specify via dialog  FilterObject=Hm_biquad
  Out : Outport
  wires:
  Generated Filter Block/1 -> Out/1
  In/1 -> Generated Filter Block/1

== system playback_data/Control1/Actuator Control with Torque SEA commands/Lowpass Filter1 ==
  In : Inport
  Generated Filter Block : dsparch4/Biquad Filter  Tag=BlockMethodSubSystem  IIRFiltStruct=Direct form II  CoeffSource=Specify via dialog  BiQuadCoeffs=[1.0054190789171848 -2 1.0054190789171853 1 -1.9557970115108714 0.95685429506963915]  a0Flag=Warning  IC=0  ICnum=0  ICden=0  denAccumFracLength=30  denProdOutputFracLength=30  secondMemoryFracLength=15  roundingMode=Floor  overflowMode=off  ScaleValues=[0.0010519560093213882;92.733879468734756]  optimizeScaleValues=off  ScaleValueMode=Specify via input port (g)  scaleValueFracLength=14  FilterSource=Specify via dialog  FilterObject=Hm_biquad
  Out : Outport
  wires:
  In/1 -> Generated Filter Block/1
  Generated Filter Block/1 -> Out/1

== system playback_data/Control1/Actuator Control with Torque SEA commands/Lowpass Filter2 ==
  In : Inport
  Generated Filter Block : dsparch4/Biquad Filter  Tag=BlockMethodSubSystem  IIRFiltStruct=Direct form II  CoeffSource=Specify via dialog  BiQuadCoeffs=[0.42638734887522584 0.71004939850960869 0.42638734887522595 1 0.054295561672899631 0.19751119790393634]  a0Flag=Warning  IC=0  ICnum=0  ICden=0  denAccumFracLength=30  denProdOutputFracLength=30  secondMemoryFracLength=15  roundingMode=Floor  overflowMode=off  ScaleValues=[0.80099018345858064;1]  optimizeScaleValues=off  ScaleValueMode=Specify via input port (g)  scaleValueFracLength=14  FilterSource=Specify via dialog  FilterObject=Hm_biquad
  Out : Outport
  wires:
  In/1 -> Generated Filter Block/1
  Generated Filter Block/1 -> Out/1

== system playback_data/Control1/Actuator Control with Torque SEA commands/Lowpass Filter5 ==
  In : Inport
  Generated Filter Block : dsparch4/Biquad Filter  Tag=BlockMethodSubSystem  IIRFiltStruct=Direct form II  CoeffSource=Specify via dialog  BiQuadCoeffs=[1.0054190789171848 -2 1.0054190789171853 1 -1.9557970115108714 0.95685429506963915]  a0Flag=Warning  IC=0  ICnum=0  ICden=0  denAccumFracLength=30  denProdOutputFracLength=30  secondMemoryFracLength=15  roundingMode=Floor  overflowMode=off  ScaleValues=[0.0010519560093213882;92.733879468734756]  optimizeScaleValues=off  ScaleValueMode=Specify via input port (g)  scaleValueFracLength=14  FilterSource=Specify via dialog  FilterObject=Hm_biquad
  Out : Outport
  wires:
  In/1 -> Generated Filter Block/1
  Generated Filter Block/1 -> Out/1

== system playback_data/Control1/Actuator Control with Torque SEA commands/Lowpass Filter6 ==
  In : Inport
  Generated Filter Block : dsparch4/Biquad Filter  Tag=BlockMethodSubSystem  IIRFiltStruct=Direct form II  CoeffSource=Specify via dialog  BiQuadCoeffs=[1.0054190789171848 -2 1.0054190789171853 1 -1.9557970115108714 0.95685429506963915]  a0Flag=Warning  IC=0  ICnum=0  ICden=0  denAccumFracLength=30  denProdOutputFracLength=30  secondMemoryFracLength=15  roundingMode=Floor  overflowMode=off  ScaleValues=[0.0010519560093213882;92.733879468734756]  optimizeScaleValues=off  ScaleValueMode=Specify via input port (g)  scaleValueFracLength=14  FilterSource=Specify via dialog  FilterObject=Hm_biquad
  Out : Outport
  wires:
  Generated Filter Block/1 -> Out/1
  In/1 -> Generated Filter Block/1

== system playback_data/Control1/Actuator Control with Torque SEA commands/Measured Forces on Foot ==
  R/L Leg Length [m] x2 : Inport
  R/L Leg Width [m] x2 : Inport  Port=2
  Torques on Load [Nm] x4 : Inport  Port=3
  Divide : Product  Inputs=/*
  Divide1 : Product  Inputs=/*
  Gain3 : Gain  Gain=-1
  Gain6 : Gain  Gain=-1
  Selector2 : Selector  InputPortWidth=4  Indices=[1 3]
  Selector7 : Selector  InputPortWidth=4  Indices=[2 4]
  Sum5 : Sum  Inputs=|-+
  Sum6 : Sum  Inputs=++|
  R/L Orthogonal Force [N] x2 : Outport
  R/L Axial Force [N] x2 : Outport  Port=2
  wires:
  Divide/1 -> Gain6/1
  R/L Leg Length [m] x2/1 -> Divide/1
  R/L Leg Width [m] x2/1 -> Divide1/1
  Torques on Load [Nm] x4/1 -> Selector7/1, Selector2/1
  Divide1/1 -> Gain3/1
  Selector2/1 -> Sum6/1, Sum5/1
  Sum6/1 -> Divide/2
  Selector7/1 -> Sum5/2, Sum6/2
  Sum5/1 -> Divide1/2
  Gain3/1 -> R/L Axial Force [N] x2/1
  Gain6/1 -> R/L Orthogonal Force [N] x2/1

== system playback_data/Control1/Actuator Control with Torque SEA commands/SEA Controller (Torque) ==
  phi_load [rad] x4 : Inport
  phi_gear [rad] x4 : Inport  Port=2
  dphi_load [rad/s] x4 : Inport  Port=3
  dphi_gear [rad/s] x4 : Inport  Port=4
  tau_des sagittal [Nm] x4 : Inport  Port=5
  dtau_des sagittal [Nm] x4 : Inport  Port=6
  Abs : Abs
  Antiresonance Compensation : Subsystem
  Friction Compensation : Subsystem
  Loaded Unloaded Switch : Subsystem
  P gain ramp : Lookup_n-D  NumberOfTableDimensions=1  BreakpointsForDimension1=[0,65,350,700]  Table=0.60*[0.3, 0.3, 6.0, 6.0]  InternalRulePriority=Speed  RndMeth=Simplest  InputSameDT=on
  Product : Product  SampleTime=sample_time  RndMeth=Zero
  Product2 : Product  RndMeth=Zero
  Spring Stiffness : Gain  Gain=k_sea_low
  Spring Stiffness 1 : Gain  Gain=k_sea_low
  Sum1 : Sum  Inputs=-+|
  Sum10 : Sum  Inputs=|++
  Sum2 : Sum  Inputs=|+-
  Sum3 : Sum  Inputs=++|
  Sum5 : Sum  Inputs=|+-
  Sum6 : Sum  Inputs=-+|
  Sum7 : Sum  Inputs=+|+
  Torque Limiter (outside) 1 : Saturate  UpperLimit=max_sagittal_loaded_torque  LowerLimit=-max_sagittal_loaded_torque
      settings: AttributesFormatString=Hi: %<UpperLimit>\nLo: %<LowerLimit>
  Torque Limiter (outside) 3 : Saturate  UpperLimit=max_sagittal_unloaded_torque  LowerLimit=-max_sagittal_unloaded_torque
      settings: AttributesFormatString=Hi: %<UpperLimit>\nLo: %<LowerLimit>
  Torque Threshold : simulink/Logic and Bit Operations/Compare To Constant  relop=>=  const=loaded_unloaded_torque_threshold  OutDataTypeStr=boolean
  critical damping : Subsystem
  tau_cmd sagittal [Nm] x4 : Outport
  tau_measured [Nm] x4 : Outport  Port=2
  wires:
  Product2/1 -> Sum7/2
  Sum2/1 -> Product2/2
  Sum5/1 -> Product/2
  dphi_gear [rad/s] x4/1 -> Friction Compensation/1(Motor Velocity [rad/s]), Sum6/2
  dphi_load [rad/s] x4/1 -> Sum6/1
  Spring Stiffness 1/1 -> Sum2/2
  Sum6/1 -> Spring Stiffness 1/1
  dtau_des sagittal [Nm] x4/1 -> Sum2/1
  tau_des sagittal [Nm] x4/1 -> Sum5/1
  phi_gear [rad] x4/1 -> Sum1/2
  phi_load [rad] x4/1 -> Sum1/1
  Sum1/1 -> Spring Stiffness/1
  Spring Stiffness/1 -> Sum3/1, Sum5/2, Abs/1, tau_measured [Nm] x4/1
  Sum10/1 -> Antiresonance Compensation/1(Torque), Torque Limiter (outside) 1/1
  P gain ramp/1 -> critical damping/1(p gain), Product/1
  Product/1 -> Sum7/1
  Sum7/1 -> Sum3/2
  Torque Limiter (outside) 1/1 -> Loaded Unloaded Switch/1(Loaded Signal)
  Torque Limiter (outside) 3/1 -> Loaded Unloaded Switch/2(Unloaded Signal)
  Antiresonance Compensation/1(Filtered Torque) -> Torque Limiter (outside) 3/1
  Friction Compensation/1(Friction Compensation [Nm]) -> Sum10/2
  Loaded Unloaded Switch/1(Signal) -> tau_cmd sagittal [Nm] x4/1
  Torque Threshold/1 -> Loaded Unloaded Switch/3(Loaded/Unloaded [1/0] x4)
  Abs/1 -> P gain ramp/1, Torque Threshold/1
  Sum3/1 -> Sum10/1
  critical damping/1(d gain) -> Product2/1

== system playback_data/Control1/Actuator Control with Torque SEA commands/SEA Controller (Velocity) ==
  phi_load [rad] x4 : Inport
  phi_gear [rad] x4 : Inport  Port=2
  dphi_load [rad/s] x4 : Inport  Port=3
  tau_des sagittal [Nm] x4 : Inport  Port=4
  dtau_des sagittal [Nm] x4 : Inport  Port=5
  Reset SEA Control [1/0] x4 : Inport  Port=6
  Stance (1) or Swing (0) x4 : Inport  Port=7
  Demux : Demux
  Demux1 : Demux
  Demux2 : Demux
  Feedback : Scope  NumInputPorts=4
      settings: YMin=-4~-0.9~-5~-5  YMax=4.5~1~5~5  SaveName=ScopeData7  SampleInput=on
  Feedforward : Scope  NumInputPorts=4
      settings: YMin=-4~-0.9~-5~-5  YMax=4.5~1~5~5  SaveName=ScopeData4  SampleInput=on
  Gain3 : Gain  Gain=1./k_sea_low
  Integrator : Subsystem
  Kp : Constant  Value=0.016
  Lowpass Filter (Stance) : Subsystem  DialogController=fdesignblkfcn  InitFcn=fdesignblkfcn(gcbh, {'InitFcn'});  mask(Lowpass Filter){}
      mask help: Design a lowpass filter
      settings: CopyFcn=fdesignblkfcn(gcbh, {'CopyFcn'});
      mask Help: helpview(mapfilelocation('dsp'), 'dsplowpassfilter');
      mask Display: disp('Lowpass')
  Lowpass Filter (Swing) : Subsystem  DialogController=fdesignblkfcn  InitFcn=fdesignblkfcn(gcbh, {'InitFcn'});  mask(Lowpass Filter){}
      mask help: Design a lowpass filter
      settings: CopyFcn=fdesignblkfcn(gcbh, {'CopyFcn'});
      mask Help: helpview(mapfilelocation('dsp'), 'dsplowpassfilter');
      mask Display: disp('Lowpass')
  Nonlinear Spring Force : MATLAB Function  TreatAsAtomicUnit=on
  Product : Product
  Stance Swing : Scope  NumInputPorts=4
      settings: YMin=-4~-0.9~-5~-5  YMax=4.5~1~5~5  SaveName=ScopeData5  SampleInput=on
  Stance or Swing : Subsystem
  Stance or Swing1 : Subsystem
  Stance or Swing2 : Subsystem
  Sum1 : Sum  Inputs=-+|
  Sum10 : Sum  Inputs=++|
  Sum4 : Sum  Inputs=|++
  Sum5 : Sum  Inputs=|+-
  Sum6 : Sum  Inputs=|++
  Ti : Gain  Gain=1/0.150
  Torque Limiter (stance) : Saturate  UpperLimit=700  LowerLimit=-700
      settings: AttributesFormatString=Hi: %<UpperLimit>\nLo: %<LowerLimit>
  Torque Limiter (swing) : Saturate  UpperLimit=80  LowerLimit=-80
      settings: AttributesFormatString=Hi: %<UpperLimit>\nLo: %<LowerLimit>
  Velocity Notch Filter (Swing) : dspfdesign/Notch-Peak Filter  Specification=Quality factor and center frequency  Bandwidth=27  QualityFactor=2.5  CenterFrequency=27  BandwidthCoefficient=0.72654  CenterFrequencyCoefficient=0  Output=Notch  InheritSampleRate=off  SampleRate=update_freq  SimulateUsing=Code generation
  Velocity Command [rad/s] x4 : Outport  PortDimensions=4
  tau_measured [Nm] x4 : Outport  Port=2
  wires:
  Sum1/1 -> Nonlinear Spring Force/1(deflections)
  Nonlinear Spring Force/1(tau_sea) -> tau_measured [Nm] x4/1, Sum5/2
  Product/1 -> Ti/1, Sum10/1
  Sum6/1 -> Stance or Swing1/2(Signal True x4), Velocity Notch Filter (Swing)/1
  Gain3/1 -> Sum4/1
  dtau_des sagittal [Nm] x4/1 -> Gain3/1
  Reset SEA Control [1/0] x4/1 -> Integrator/2(Reset [1/0])
  Sum5/1 -> Product/1
  Integrator/1(Integrated) -> Sum10/2
  Ti/1 -> Integrator/1(Signal)
  dphi_load [rad/s] x4/1 -> Sum4/2
  Sum4/1 -> Lowpass Filter (Stance)/1(In), Lowpass Filter (Swing)/1(In)
  Lowpass Filter (Stance)/1(Out) -> Stance or Swing2/2(Signal True x4), Demux1/1
  Kp/1 -> Product/2
  Stance or Swing/1(Selected x4) -> Sum5/1
  Torque Limiter (swing)/1 -> Stance or Swing/3(Signal False x4)
  Torque Limiter (stance)/1 -> Stance or Swing/2(Signal True x4)
  Stance or Swing1/1(Selected x4) -> Velocity Command [rad/s] x4/1
  Velocity Notch Filter (Swing)/1 -> Stance or Swing1/3(Signal False x4)
  Demux/4 -> Feedback/4
  Demux/3 -> Feedback/3
  Demux/2 -> Feedback/2
  Demux/1 -> Feedback/1
  Demux1/1 -> Feedforward/1
  Demux1/2 -> Feedforward/2
  Demux1/3 -> Feedforward/3
  Demux1/4 -> Feedforward/4
  tau_des sagittal [Nm] x4/1 -> Torque Limiter (stance)/1, Torque Limiter (swing)/1
  phi_gear [rad] x4/1 -> Sum1/2
  phi_load [rad] x4/1 -> Sum1/1
  Stance (1) or Swing (0) x4/1 -> Demux2/1, Stance or Swing2/1(True/False x4), Stance or Swing1/1(True/False x4), Stance or Swing/1(True/False x4)
  Demux2/3 -> Stance Swing/3
  Demux2/2 -> Stance Swing/2
  Demux2/1 -> Stance Swing/1
  Demux2/4 -> Stance Swing/4
  Sum10/1 -> Demux/1, Sum6/1
  Lowpass Filter (Swing)/1(Out) -> Stance or Swing2/3(Signal False x4)
  Stance or Swing2/1(Selected x4) -> Sum6/2

== system playback_data/Control1/Actuator Control with Torque SEA commands/Stance or Swing1 ==
  True/False x4 : Inport
  Signal True x4 : Inport  Port=2
  Signal False x4 : Inport  Port=3
  Demux : Demux
  Demux1 : Demux
  Demux2 : Demux
  Mux : Mux
  Switch{,1..3} (4 alike) : Switch  Criteria=u2 ~= 0
  Selected x4 : Outport
  wires:
  Switch3/1 -> Mux/4
  Switch2/1 -> Mux/3
  Switch1/1 -> Mux/2
  Switch/1 -> Mux/1
  Demux1/4 -> Switch3/2
  Demux1/3 -> Switch2/2
  Demux1/2 -> Switch1/2
  Demux1/1 -> Switch/2
  Demux2/4 -> Switch3/3
  Demux2/3 -> Switch2/3
  Demux2/2 -> Switch1/3
  Demux2/1 -> Switch/3
  Demux/4 -> Switch3/1
  Demux/3 -> Switch2/1
  Demux/2 -> Switch1/1
  Demux/1 -> Switch/1
  Signal False x4/1 -> Demux2/1
  Signal True x4/1 -> Demux/1
  True/False x4/1 -> Demux1/1
  Mux/1 -> Selected x4/1
